simulink model "WT_pitch_actuator_no_sat"  (R2024a)
settings: Solver=FixedStepAuto  StartTime=0.0  StopTime=0.8  FixedStep=0.001  RelTol=1e-3
settings Model: Creator=ml4  LastModifiedBy=ml4
settings RTWCC: GenCodeOnly=on  GenerateMakefile=off  PackageGeneratedCodeAndArtifacts=on
settings GRTTargetCC: RTWCAPISignals=on  RTWCAPIParams=on  RTWCAPIStates=on  RTWCAPIRootIO=on

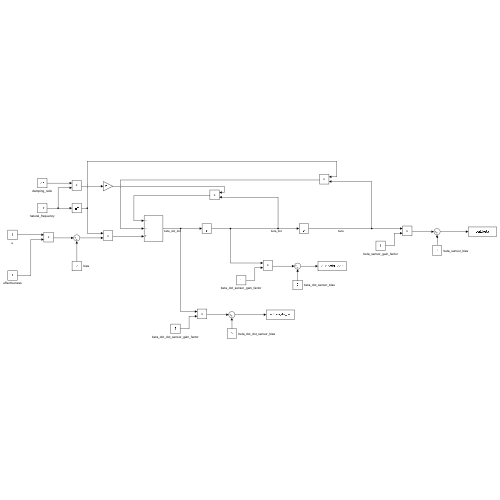
[thumbnail: Simulink's stored preview of the top-level diagram]
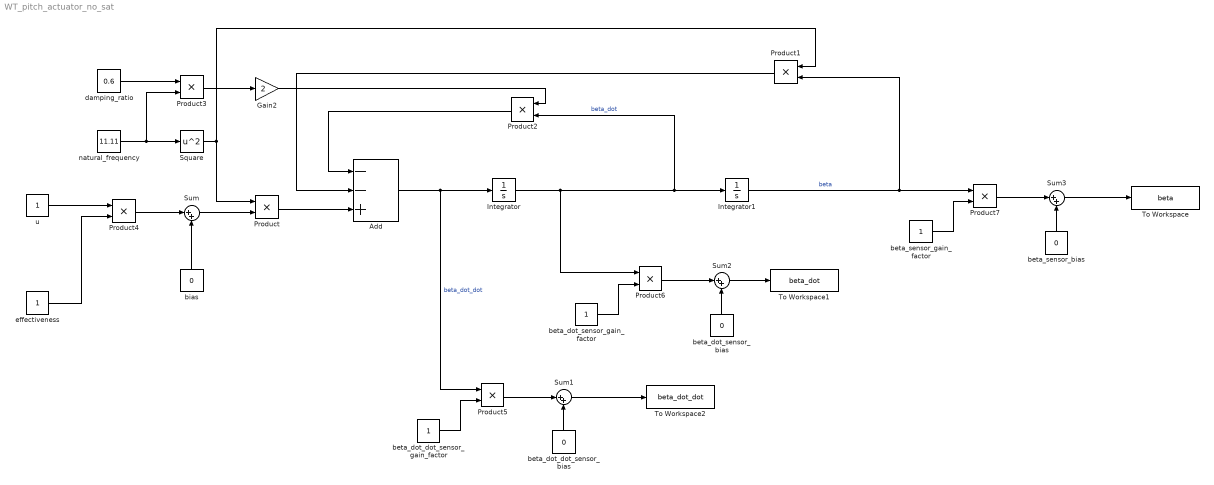
== system WT_pitch_actuator_no_sat ==
  Add : Sum  Inputs=--+
  Gain2 : Gain  Gain=2
  Integrator : Integrator
  Integrator1 : Integrator
  Product{,1..7} (8 alike) : Product
  Square : Math  Operator=square
  Sum{,1..3} (4 alike) : Sum  Inputs=|++
  To Workspace : ToWorkspace  VariableName=beta  SampleTime=-1
      settings: Save2DSignal=2-D array (concatenate along first dimension)
  To Workspace1 : ToWorkspace  VariableName=beta_dot  SampleTime=-1
      settings: Save2DSignal=2-D array (concatenate along first dimension)
  To Workspace2 : ToWorkspace  VariableName=beta_dot_dot  SampleTime=-1
      settings: Save2DSignal=2-D array (concatenate along first dimension)
  beta_dot_dot_sensor_bias : Constant  Value=0
  beta_dot_dot_sensor_gain_factor : Constant
  beta_dot_sensor_bias : Constant  Value=0
  beta_dot_sensor_gain_factor : Constant
  beta_sensor_bias : Constant  Value=0
  beta_sensor_gain_factor : Constant
  bias : Constant  Value=0
  damping_ratio : Constant  Value=0.6
  effectiveness : Constant
  natural_frequency : Constant  Value=11.11
  u : Constant
  wires:
  Product1/1 -> Add/2
  Gain2/1 -> Product2/1
  damping_ratio/1 -> Product3/1
  Square/1 -> Product1/1, Product/1
  Sum/1 -> Product/2
  natural_frequency/1 -> Product3/2, Square/1
  bias/1 -> Sum/2
  Product4/1 -> Sum/1
  Integrator/1 -> Product2/2, Integrator1/1, Product6/1  "beta_dot"
  Add/1 -> Integrator/1, Product5/1  "beta_dot_dot"
  Product2/1 -> Add/1
  Product/1 -> Add/3
  u/1 -> Product4/1
  Product3/1 -> Gain2/1
  Integrator1/1 -> Product7/1, Product1/2  "beta"
  Product5/1 -> Sum1/1
  Sum1/1 -> To Workspace2/1
  effectiveness/1 -> Product4/2
  beta_dot_dot_sensor_gain_factor/1 -> Product5/2
  beta_dot_dot_sensor_bias/1 -> Sum1/2
  Product6/1 -> Sum2/1
  beta_dot_sensor_gain_factor/1 -> Product6/2
  beta_dot_sensor_bias/1 -> Sum2/2
  Sum2/1 -> To Workspace1/1
  Product7/1 -> Sum3/1
  beta_sensor_gain_factor/1 -> Product7/2
  beta_sensor_bias/1 -> Sum3/2
  Sum3/1 -> To Workspace/1
